simulink model "CD_head_modal_ws"  (R2015a)
settings: Solver=ode23tb  StartTime=0.0  StopTime=10.0  RelTol=1e-3
values from neighbouring files (symbols this model uses):
  CC = 2*zeta*sqrt(MM.*KK)    [CD_head_modal.m]
  KK = diag(KK)    [CD_head_modal.m]
  MM = diag(MM)    [CD_head_modal.m]
undefined symbols (not defined in the file or in its folder): V
settings Model: Creator=ron  LastModifiedBy=ron
settings DebuggingCC: UnderspecifiedInitializationDetection=Classic  MergeDetectMultiDrivingBlocksExec=none  SolverPrmCheckMsg=warning

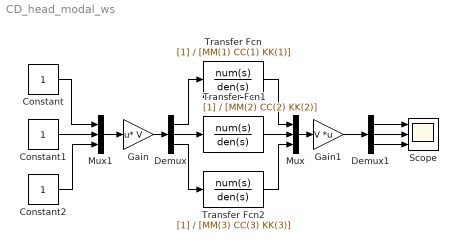
== system CD_head_modal_ws ==
  Constant : Constant
  Constant1 : Constant
  Constant2 : Constant
  Demux : Demux  Outputs=3
  Demux1 : Demux  Outputs=3
  Gain : Gain  Gain=V  Multiplication=Matrix(u*K)
  Gain1 : Gain  Gain=V  Multiplication=Matrix(K*u)
  Mux : Mux  Inputs=3
  Mux1 : Mux  Inputs=3
  Scope : Scope  NumInputPorts=3
      settings: YMin=-5~-5~-5  YMax=5~5~5
  Transfer Fcn : TransferFcn  Denominator=[MM(1) CC(1) KK(1)]
  Transfer Fcn1 : TransferFcn  Denominator=[MM(2) CC(2) KK(2)]
  Transfer Fcn2 : TransferFcn  Denominator=[MM(3) CC(3) KK(3)]
  wires:
  Mux/1 -> Gain1/1
  Transfer Fcn/1 -> Mux/1
  Transfer Fcn1/1 -> Mux/2
  Transfer Fcn2/1 -> Mux/3
  Demux/1 -> Transfer Fcn/1
  Demux/2 -> Transfer Fcn1/1
  Demux/3 -> Transfer Fcn2/1
  Gain/1 -> Demux/1
  Gain1/1 -> Demux1/1
  Mux1/1 -> Gain/1
  Constant1/1 -> Mux1/2
  Constant/1 -> Mux1/1
  Constant2/1 -> Mux1/3
  Demux1/1 -> Scope/1
  Demux1/2 -> Scope/2
  Demux1/3 -> Scope/3
